simulink library "csu_ppd_phase_plane_distance_lib"  (R2014b)
settings: Solver=ode45  StartTime=0.0  StopTime=10.0  RelTol=1e-3
undefined symbols (not defined in the file or in its folder): csc_cnt_dt
libraries: simulink x4, util_info_lib x1
settings Model: Creator=Nilesh  LastModifiedBy=mstewart

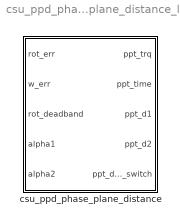
== system csu_ppd_phase_plane_distance_lib ==
  csu_ppd_phase_plane_distance : Subsystem

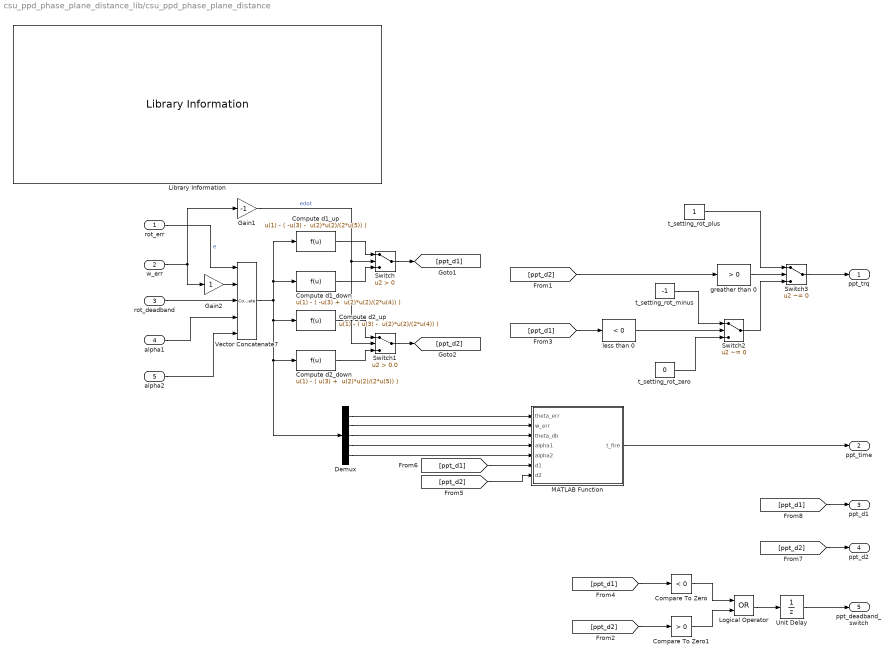
== system csu_ppd_phase_plane_distance_lib/csu_ppd_phase_plane_distance ==
  rot_err : Inport
  w_err : Inport  Port=2
  rot_deadband : Inport  Port=3
  alpha1 : Inport  Port=4
  alpha2 : Inport  Port=5
  Compare To Zero : simulink/Logic and Bit Operations/Compare To Zero  relop=<  OutDataTypeStr=uint8  ZeroCross=off
  Compare To Zero1 : simulink/Logic and Bit Operations/Compare To Zero  relop=>  OutDataTypeStr=uint8  ZeroCross=off
  Compute d1_down : Fcn  Expr="u(1) - ( -u(3) +  u(2)*u(2)/(2*u(4)) )"
  Compute d1_up : Fcn  Expr="u(1) - ( -u(3) -  u(2)*u(2)/(2*u(5)) )"
  Compute d2_down : Fcn  Expr="u(1) - ( u(3) +  u(2)*u(2)/(2*u(5)) )"
  Compute d2_up : Fcn  Expr="u(1) - ( u(3) -  u(2)*u(2)/(2*u(4)) )"
  Demux : Demux  Outputs=5
  Gain1 : Gain  Gain=-1
  Gain2 : Gain
  Library Information : util_info_lib/Library Information  owner='NONE'
  Logical Operator : Logic  Operator=OR  AllPortsSameDT=off  OutDataTypeStr=boolean
  MATLAB Function : MATLAB Function  TreatAsAtomicUnit=on
  Switch : Switch  Criteria=u2 > Threshold
  Switch1 : Switch  Criteria=u2 > Threshold  Threshold=0.0
  Switch2 : Switch  Criteria=u2 ~= 0
  Switch3 : Switch  Criteria=u2 ~= 0
  Unit Delay : UnitDelay  SampleTime=csc_cnt_dt
  Vector Concatenate7 : Concatenate  NumInputs=5
  greather than 0 : simulink/Logic and Bit Operations/Compare To Constant  relop=>  const=0  OutDataTypeStr=uint8  ZeroCross=off
  less than 0 : simulink/Logic and Bit Operations/Compare To Constant  relop=<  const=0  OutDataTypeStr=uint8  ZeroCross=off
  t_setting_rot_minus : Constant  Value=-1  OutDataTypeStr=int8
  t_setting_rot_plus : Constant  OutDataTypeStr=int8
  t_setting_rot_zero : Constant  Value=0  OutDataTypeStr=int8
  ppt_trq : Outport
  ppt_time : Outport  Port=2
  ppt_d1 : Outport  Port=3
  ppt_d2 : Outport  Port=4
  ppt_deadband_switch : Outport  Port=5
  wires:
  Switch1/1 -> [ppt_d2]
  Switch/1 -> [ppt_d1]
  Compute d2_down/1 -> Switch1/3
  Compute d2_up/1 -> Switch1/1
  Compute d1_down/1 -> Switch/3
  Compute d1_up/1 -> Switch/1
  Vector Concatenate7/1 -> Demux/1, Compute d2_down/1, Compute d2_up/1, Compute d1_up/1, Compute d1_down/1
  alpha2/1 -> Vector Concatenate7/5
  alpha1/1 -> Vector Concatenate7/4
  rot_deadband/1 -> Vector Concatenate7/3
  rot_err/1 -> Vector Concatenate7/1  "e"
  greather than 0/1 -> Switch3/2
  less than 0/1 -> Switch2/2
  Switch2/1 -> Switch3/3
  t_setting_rot_plus/1 -> Switch3/1
  t_setting_rot_zero/1 -> Switch2/3
  t_setting_rot_minus/1 -> Switch2/1
  Switch3/1 -> ppt_trq/1
  [ppt_d1] -> Compare To Zero/1
  [ppt_d2] -> Compare To Zero1/1
  Compare To Zero/1 -> Logical Operator/1
  Compare To Zero1/1 -> Logical Operator/2
  Logical Operator/1 -> Unit Delay/1
  Unit Delay/1 -> ppt_deadband_switch/1
  MATLAB Function/1(t_fire) -> ppt_time/1
  [ppt_d2] -> MATLAB Function/7(d2)
  [ppt_d1] -> MATLAB Function/6(d1)
  Demux/1 -> MATLAB Function/1(theta_err)
  Demux/2 -> MATLAB Function/2(w_err)
  Demux/3 -> MATLAB Function/3(theta_db)
  Demux/4 -> MATLAB Function/4(alpha1)
  Demux/5 -> MATLAB Function/5(alpha2)
  [ppt_d2] -> greather than 0/1
  [ppt_d1] -> less than 0/1
  [ppt_d1] -> ppt_d1/1
  [ppt_d2] -> ppt_d2/1
  w_err/1 -> Gain2/1, Gain1/1
  Gain1/1 -> Switch1/2, Switch/2  "edot"
  Gain2/1 -> Vector Concatenate7/2

== matlab function csu_ppd_phase_plane_distance_lib/csu_ppd_phase_plane_distance/MATLAB Function ==
  data: theta_err input; w_err input; theta_db input; alpha1 input; alpha2 input; t_fire output; d1 input; d2 input
function t_fire = fcn(theta_err,w_err,theta_db,alpha1,alpha2,d1,d2)
%#codegen


w_err = -w_err; %-u(2);


if d1 < 0
   
    t_fire = (1/alpha1)*(sqrt( (alpha2/(alpha1 + alpha2))*(2*alpha1*theta_db -2*alpha1*theta_err + w_err*w_err) ) - w_err);

    
elseif d2 > 0
    
%     t_fire = (1/alpha1)*(sqrt( (alpha2/(alpha1 + alpha2))*(-2*alpha1*theta_db +2*alpha1*theta_err + w_err*w_err) ) + w_err);
    t_fire = (1/alpha1)*(sqrt( (alpha2/(alpha1 + alpha2))*(2*alpha1*theta_db +2*alpha1*theta_err + w_err*w_err) ) + w_err);
    
else
    
    t_fire = 0;
    
end
